simulink model "Embeddedsystem_Simulink"  (R2020a)
settings: Solver=FixedStepDiscrete  StartTime=0.0  StopTime=inf  FixedStep=0.1  RelTol=1e-3  EnableMultiTasking=on
libraries: frdmk64flib x4, simulink_extras x3, dspstat3 x1
settings Model: SimulationMode=external  ExtModeTrigDuration=5  Creator=luca9  LastModifiedBy=luca9
settings OptimizationCC: EnhancedBackFolding=on  PassReuseOutputArgsAs=Individual arguments  ZeroExternalMemoryAtStartup=off  ZeroInternalMemoryAtStartup=off  MaxStackSize=64  OptimizeBlockOrder=speed  DifferentSizesBufferReuse=on  OptimizationCustomize=off  EfficientTunableParamExpr=on
settings DebuggingCC: ParameterTunabilityLossMsg=error
settings HardwareCC: ProdBitPerPointer=32  ProdBitPerSizeT=32  ProdBitPerPtrDiffT=32  ProdLargestAtomicInteger=Long  ProdLargestAtomicFloat=Double  ProdWordSize=32  ProdHWDeviceType=ARM Compatible->ARM Cortex
settings SFSimCC: MATLABDynamicMemAlloc=off
settings RTWCC: SystemTargetFile=ert.tlc  HardwareBoard=NXP FRDM-K64F  TemplateMakefile=ert_default_tmf  GenerateReport=on  Toolchain=GNU Tools for ARM Embedded Processors
settings CodeAppCC: ForceParamTrailComments=on  IgnoreCustomStorageClasses=off  OperatorAnnotations=on  SimulinkDataObjDesc=on  SFDataObjDesc=on  InsertBlockDesc=on
settings ERTTargetCC: ExtMode=on  ExtModeTransport=4  ExtModeMexFile=sendToCommService  ExtModeMexArgs='sim_finalassignment' 0

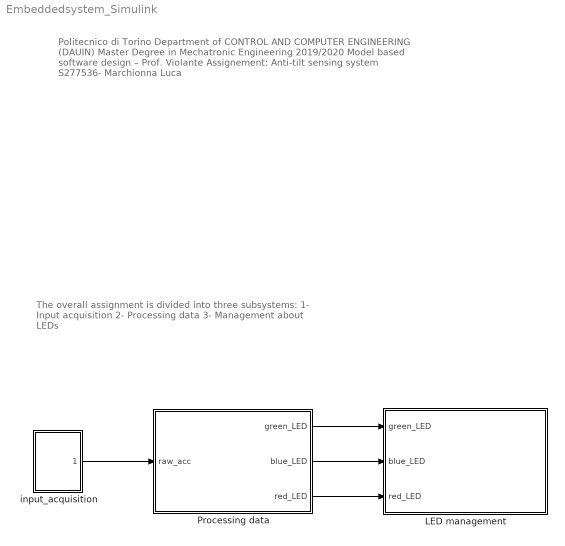
== system Embeddedsystem_Simulink ==
  note: The overall assignment is divided into three subsystems:
      | 1- Input acquisition
      | 2- Processing data
      | 3- Management about LEDs
  note: Politecnico di Torino
      | Department of CONTROL AND COMPUTER ENGINEERING (DAUIN)
      | Master Degree in Mechatronic Engineering
      | 2019/2020
      |
      | Model based software design – Prof. Violante
      | Assignement: Anti-tilt sensing system
      | S277536- Marchionna Luca
  " LED management" : Subsystem
  Processing data : Subsystem
  input_acquisition : Subsystem
  wires:
  input_acquisition/1(raw_acc) -> Processing data/1(raw_acc)
  Processing data/1(green_LED) -> " LED management"/1(green_LED)
  Processing data/2(blue_LED) -> " LED management"/2(blue_LED)
  Processing data/3(red_LED) -> " LED management"/3(red_LED)

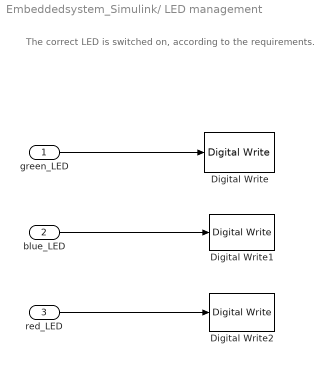
== system Embeddedsystem_Simulink/ LED management ==
  note: The correct LED is switched on, according to the requirements.
  green_LED : Inport
  blue_LED : Inport  Port=2
  red_LED : Inport  Port=3
  Digital Write : frdmk64flib/Digital Write  Whichpin=GREEN_LED
  Digital Write1 : frdmk64flib/Digital Write  Whichpin=BLUE_LED
  Digital Write2 : frdmk64flib/Digital Write  Whichpin=RED_LED
  wires:
  green_LED/1 -> Digital Write/1
  blue_LED/1 -> Digital Write1/1
  red_LED/1 -> Digital Write2/1

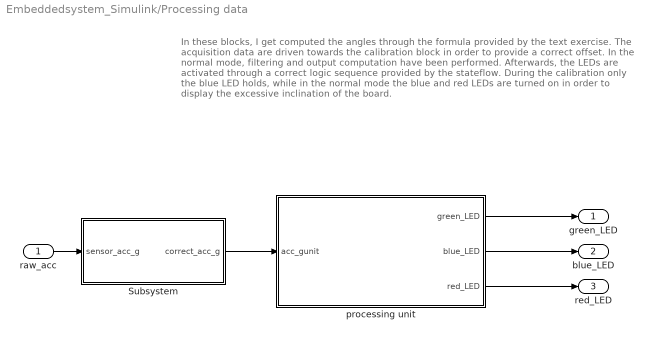
== system Embeddedsystem_Simulink/Processing data ==
  note: In these blocks, I get computed the angles through the formula provided by the text exercise. The acquisition data are driven towards the calibration block in order to provide a correct offset. In the normal mode, filtering and output computation have been performed.
      | Afterwards, the LEDs are activated through a correct logic sequence provided by the stateflow. During the calibration only the blue LED holds, while in the normal mode the blue and red LEDs are turned on in order to display the excessive inclination of the board.
  raw_acc : Inport
  Subsystem : Subsystem
  processing unit : Subsystem
  green_LED : Outport
  blue_LED : Outport  Port=2
  red_LED : Outport  Port=3
  wires:
  raw_acc/1 -> Subsystem/1(sensor_acc_g)
  Subsystem/1(correct_acc_g) -> processing unit/1(acc_gunit)
  processing unit/1(green_LED) -> green_LED/1
  processing unit/2(blue_LED) -> blue_LED/1
  processing unit/3(red_LED) -> red_LED/1

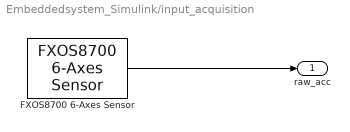
== system Embeddedsystem_Simulink/input_acquisition ==
  FXOS8700 6-Axes Sensor : frdmk64flib/FXOS8700 6-Axes Sensor  Activesensor=Accelerometer only  ODR=50Hz  HybridODR=400Hz  Accelfullrange=-2g to +2g  SampleTime=-1
  raw_acc : Outport
  wires:
  FXOS8700 6-Axes Sensor/1 -> raw_acc/1

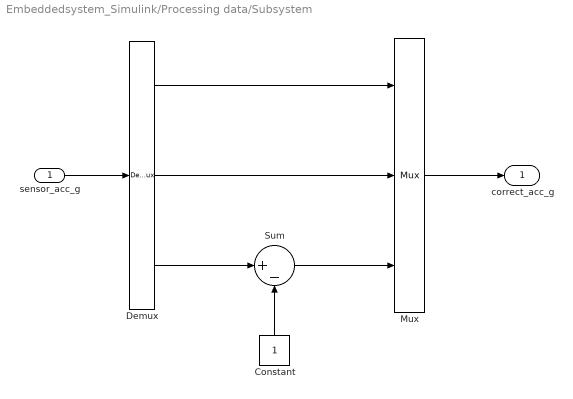
== system Embeddedsystem_Simulink/Processing data/Subsystem ==
  sensor_acc_g : Inport
  Constant : Constant
  Demux : Demux  Outputs=3
  Mux : Mux  Inputs=3
  Sum : Sum  Inputs=|+-
  correct_acc_g : Outport
  wires:
  sensor_acc_g/1 -> Demux/1
  Demux/3 -> Sum/1
  Mux/1 -> correct_acc_g/1
  Constant/1 -> Sum/2
  Demux/2 -> Mux/2
  Demux/1 -> Mux/1
  Sum/1 -> Mux/3

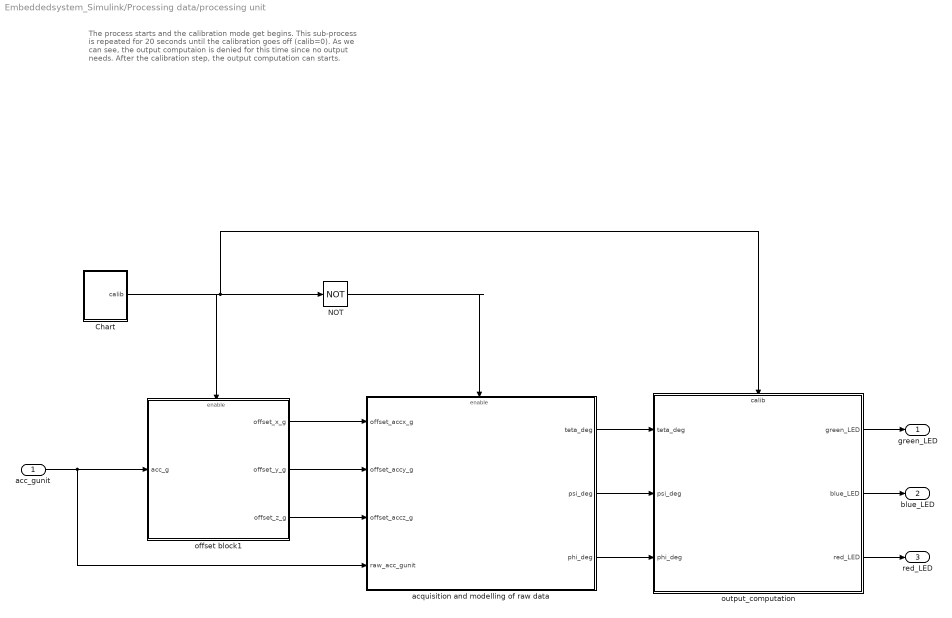
== system Embeddedsystem_Simulink/Processing data/processing unit ==
  note: The process starts and the calibration mode get begins. This sub-process is repeated for 20 seconds until the calibration goes off (calib=0). As we can see, the output computaion is denied for this time since no output needs. After the calibration step, the output computation can starts.
  acc_gunit : Inport
  Chart : Stateflow chart  TreatAsAtomicUnit=on
      settings: PortSchema="{\"entries\":[{\"content\":{\"sides\":[{\"content\":{\"connectorIds\":[]},\"type\":\"ConnectorPlacement.EquallySpacedRectSide\",\"uuid\":\"849f233e-f388-4235-a763-39289e6833f4\"},{\"content\":{\"connectorIds\":[],\"side\":\"RIGHT\"},\"type\":\"ConnectorPlacement.EquallySpacedRectSide\",\"uuid\":\"02f40bd9-b98f-494b-865f-ff408e26e3ae\"},{\"content\":{\"connectorIds\":[\"Out1\"],\"side\":\"TOP\"},\"type\":\"ConnectorPlacement.EquallySpacedRectSide\",\"uuid\":\"24d40e34-9a61-441c-a62a-e59ff23fe97d\"}]},\"type\":\"ConnectorPlacement.EquallySpacedConnector\",\"uuid\":\"996c4ffd-b183-49ea-a222-3899ee3ed888\"}],\"packageUris\":[\"http://schema.mathworks.com/mf0/Connector/19700101\"],\"version\":\"1.0\"}"
  NOT : Logic  Operator=NOT  IconShape=distinctive  AllPortsSameDT=off  OutDataTypeStr=boolean
  acquisition and modelling of raw data : Subsystem
  offset block1 : Subsystem
  output_computation : Subsystem
      settings: PortSchema="{\"entries\":[{\"content\":{\"sides\":[{\"content\":{\"connectorIds\":[\"In1\",\"In2\",\"In3\"]},\"type\":\"ConnectorPlacement.EquallySpacedRectSide\",\"uuid\":\"60aea4be-a06d-4eda-a7bc-981b750d10d1\"},{\"content\":{\"connectorIds\":[\"Out1\",\"Out2\",\"Out3\"],\"side\":\"RIGHT\"},\"type\":\"ConnectorPlacement.EquallySpacedRectSide\",\"uuid\":\"1715f949-f62d-450d-8914-9423294c064a\"},{\"content\":{\"connectorIds\":[\"In4\"],\"side\":\"TOP\"},\"type\":\"ConnectorPlacement.EquallySpacedRectSide\",\"uuid\":\"7760335e-0d5c-4cba-ab90-42ab2a2902db\"}]},\"type\":\"ConnectorPlacement.EquallySpacedConnector\",\"uuid\":\"a047fbe5-0454-4ad3-85fe-5a2833169652\"}],\"packageUris\":[\"http://schema.mathworks.com/mf0/Connector/19700101\"],\"version\":\"1.0\"}"
  green_LED : Outport
  blue_LED : Outport  Port=2
  red_LED : Outport  Port=3
  wires:
  acquisition and modelling of raw data/1(teta_deg) -> output_computation/1(teta_deg)
  Chart/1(calib) -> NOT/1, output_computation/4(calib), offset block1/Enable
  NOT/1 -> acquisition and modelling of raw data/Enable
  acc_gunit/1 -> acquisition and modelling of raw data/4(raw_acc_gunit), offset block1/1(acc_g)
  offset block1/1(offset_x_g) -> acquisition and modelling of raw data/1(offset_accx_g)
  offset block1/2(offset_y_g) -> acquisition and modelling of raw data/2(offset_accy_g)
  offset block1/3(offset_z_g) -> acquisition and modelling of raw data/3(offset_accz_g)
  acquisition and modelling of raw data/2(psi_deg) -> output_computation/2(psi_deg)
  acquisition and modelling of raw data/3(phi_deg) -> output_computation/3(phi_deg)
  output_computation/2(blue_LED) -> blue_LED/1
  output_computation/3(red_LED) -> red_LED/1
  output_computation/1(green_LED) -> green_LED/1

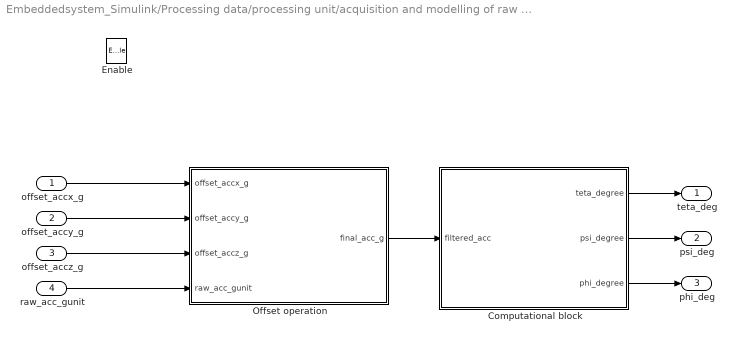
== system Embeddedsystem_Simulink/Processing data/processing unit/acquisition and modelling of raw data ==
  offset_accx_g : Inport
  offset_accy_g : Inport  Port=2
  offset_accz_g : Inport  Port=3
  raw_acc_gunit : Inport  Port=4
  Enable : EnablePort
  Computational block : Subsystem
  Offset operation : Subsystem
  teta_deg : Outport
  psi_deg : Outport  Port=2
  phi_deg : Outport  Port=3
  wires:
  offset_accx_g/1 -> Offset operation/1(offset_accx_g)
  offset_accz_g/1 -> Offset operation/3(offset_accz_g)
  Offset operation/1(final_acc_g) -> Computational block/1(filtered_acc)
  raw_acc_gunit/1 -> Offset operation/4(raw_acc_gunit)
  offset_accy_g/1 -> Offset operation/2(offset_accy_g)
  Computational block/1(teta_degree) -> teta_deg/1
  Computational block/3(phi_degree) -> phi_deg/1
  Computational block/2(psi_degree) -> psi_deg/1

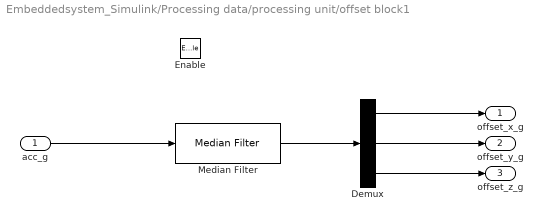
== system Embeddedsystem_Simulink/Processing data/processing unit/offset block1 ==
  acc_g : Inport
  Enable : EnablePort
  Demux : Demux  Outputs=3
  Median Filter : dspstat3/Median Filter  WindowLength=128  SimulateUsing=Interpreted execution
      settings: SourceProductBaseCode=DS
  offset_x_g : Outport
  offset_y_g : Outport  Port=2
  offset_z_g : Outport  Port=3
  wires:
  acc_g/1 -> Median Filter/1
  Demux/2 -> offset_y_g/1
  Median Filter/1 -> Demux/1
  Demux/1 -> offset_x_g/1
  Demux/3 -> offset_z_g/1

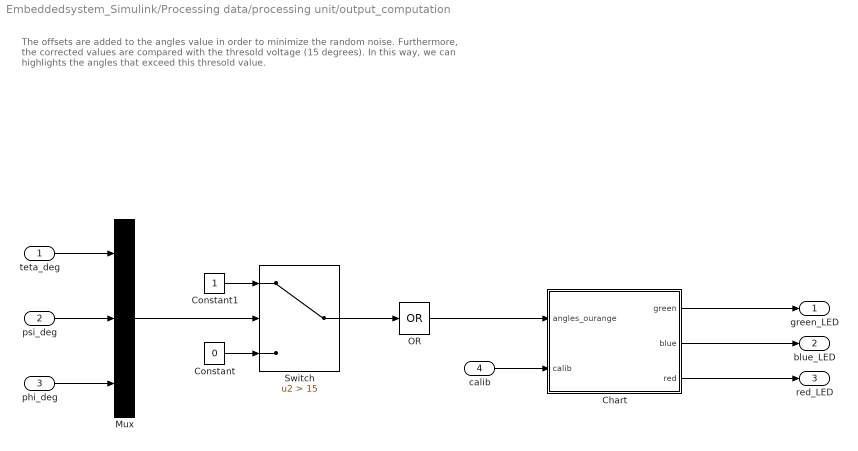
== system Embeddedsystem_Simulink/Processing data/processing unit/output_computation ==
  note: The offsets are added to the angles value in order to minimize the random noise. Furthermore, the corrected values are compared with the thresold voltage (15 degrees). In this way, we can highlights the angles that exceed this thresold value.
  teta_deg : Inport
  psi_deg : Inport  Port=2
  phi_deg : Inport  Port=3
  calib : Inport  Port=4
  Chart : Stateflow chart  TreatAsAtomicUnit=on
      settings: PortSchema="{\"entries\":[{\"content\":{\"sides\":[{\"content\":{\"connectorIds\":[\"In2\",\"In1\"]},\"type\":\"ConnectorPlacement.EquallySpacedRectSide\",\"uuid\":\"faf833d6-594c-410a-add6-5ce55fbfaff1\"},{\"content\":{\"connectorIds\":[\"Out1\",\"Out2\",\"Out3\"],\"side\":\"RIGHT\"},\"type\":\"ConnectorPlacement.EquallySpacedRectSide\",\"uuid\":\"c32c7775-d168-4cbd-91e2-7224e6ac9991\"},{\"content\":{\"connectorIds\":[],\"side\":\"TOP\"},\"type\":\"ConnectorPlacement.EquallySpacedRectSide\",\"uuid\":\"b777e44b-d9ef-458a-832d-3343b5e05232\"}]},\"type\":\"ConnectorPlacement.EquallySpacedConnector\",\"uuid\":\"539e4311-01e8-4a30-b4c5-5074bbcc3c5b\"}],\"packageUris\":[\"http://schema.mathworks.com/mf0/Connector/19700101\"],\"version\":\"1.0\"}"
  Constant : Constant  Value=0
  Constant1 : Constant
  Mux : Mux  Inputs=3
  OR : Logic  Operator=OR  Inputs=1  IconShape=distinctive  AllPortsSameDT=off  OutDataTypeStr=boolean
  Switch : Switch  Criteria=u2 > Threshold  Threshold=15
  green_LED : Outport
  blue_LED : Outport  Port=2
  red_LED : Outport  Port=3
  wires:
  Constant1/1 -> Switch/1
  Constant/1 -> Switch/3
  Switch/1 -> OR/1
  OR/1 -> Chart/2(angles_ourange)
  phi_deg/1 -> Mux/3
  psi_deg/1 -> Mux/2
  teta_deg/1 -> Mux/1
  Mux/1 -> Switch/2
  Chart/2(blue) -> blue_LED/1
  Chart/3(red) -> red_LED/1
  Chart/1(green) -> green_LED/1
  calib/1 -> Chart/1(calib)

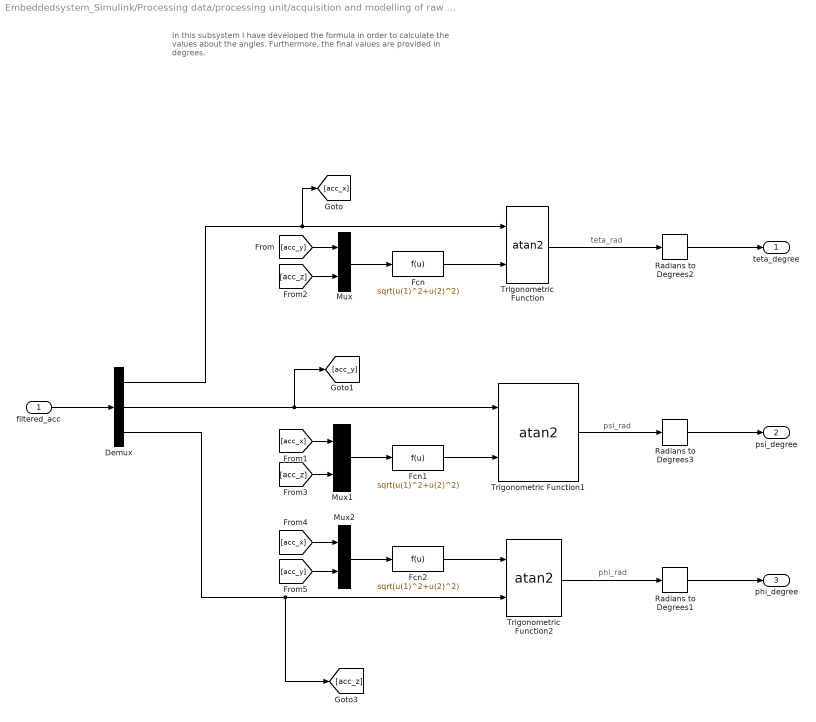
== system Embeddedsystem_Simulink/Processing data/processing unit/acquisition and modelling of raw data/Computational block ==
  note: phi_rad
  note: psi_rad
  note: teta_rad
  note: In this subsystem I have developed the formula in order to calculate the values about the angles. Furthermore, the final values are provided in degrees.
  filtered_acc : Inport
  Demux : Demux  Outputs=3
  Fcn : Fcn  Expr=sqrt(u(1)^2+u(2)^2)
  Fcn1 : Fcn  Expr=sqrt(u(1)^2+u(2)^2)
  Fcn2 : Fcn  Expr=sqrt(u(1)^2+u(2)^2)
  Mux : Mux  Inputs=2
  Mux1 : Mux  Inputs=2
  Mux2 : Mux  Inputs=2
  Radians to Degrees1 : simulink_extras/Transformations/Radians to Degrees
  Radians to Degrees2 : simulink_extras/Transformations/Radians to Degrees
  Radians to Degrees3 : simulink_extras/Transformations/Radians to Degrees
  Trigonometric Function : Trigonometry  Operator=atan2
  Trigonometric Function1 : Trigonometry  Operator=atan2
  Trigonometric Function2 : Trigonometry  Operator=atan2
  teta_degree : Outport
  psi_degree : Outport  Port=2
  phi_degree : Outport  Port=3
  wires:
  [acc_y] -> Mux2/2
  Mux/1 -> Fcn/1
  [acc_z] -> Mux1/2
  Mux1/1 -> Fcn1/1
  [acc_z] -> Mux/2
  Demux/2 -> [acc_y], Trigonometric Function1/1
  Mux2/1 -> Fcn2/1
  [acc_y] -> Mux/1
  Fcn1/1 -> Trigonometric Function1/2
  Demux/3 -> [acc_z], Trigonometric Function2/2
  [acc_x] -> Mux2/1
  [acc_x] -> Mux1/1
  Fcn2/1 -> Trigonometric Function2/1
  Fcn/1 -> Trigonometric Function/2
  Demux/1 -> [acc_x], Trigonometric Function/1
  filtered_acc/1 -> Demux/1
  Trigonometric Function/1 -> Radians to Degrees2/1
  Trigonometric Function1/1 -> Radians to Degrees3/1
  Trigonometric Function2/1 -> Radians to Degrees1/1
  Radians to Degrees2/1 -> teta_degree/1
  Radians to Degrees3/1 -> psi_degree/1
  Radians to Degrees1/1 -> phi_degree/1

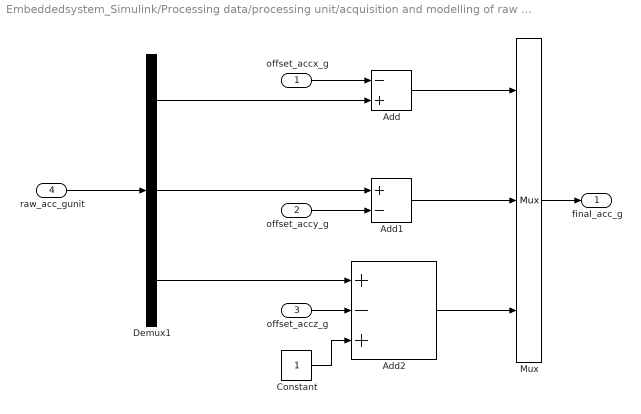
== system Embeddedsystem_Simulink/Processing data/processing unit/acquisition and modelling of raw data/Offset operation ==
  offset_accx_g : Inport
  offset_accy_g : Inport  Port=2
  offset_accz_g : Inport  Port=3
  raw_acc_gunit : Inport  Port=4
  Add : Sum  Inputs=-+
  Add1 : Sum  Inputs=+-
  Add2 : Sum  Inputs=+-+
  Constant : Constant
  Demux1 : Demux  Outputs=3
  Mux : Mux  Inputs=3
  final_acc_g : Outport
  wires:
  offset_accy_g/1 -> Add1/2
  offset_accx_g/1 -> Add/1
  offset_accz_g/1 -> Add2/2
  Demux1/2 -> Add1/1
  Demux1/3 -> Add2/1
  Demux1/1 -> Add/2
  raw_acc_gunit/1 -> Demux1/1
  Mux/1 -> final_acc_g/1
  Add1/1 -> Mux/2
  Add/1 -> Mux/1
  Constant/1 -> Add2/3
  Add2/1 -> Mux/3

== stateflow chart Embeddedsystem_Simulink/Processing data/processing unit/Chart ==
  state calibration
    en:
    calib=1;
  state calibration1
    en:
    calib=0;
  (default) -> calibration
  calibration -> calibration1 : after(20,sec)
  data: calib output

== stateflow chart Embeddedsystem_Simulink/Processing data/processing unit/output_computation/Chart ==
  state LED_inizialization
    en: blue=0;
    green=0;
    red=0;
  state LED_structureforcalibration
    en: blue=1;
    green=0;
    red=0;
  state LED_structureforinclination
    en: blue=0;
    state inclination_
      green=1;
      red=0;
    state warning1
      red=1;
      green=0;
    state no_warning
      red=0;
      green=1;
    (default) -> inclination_
    inclination_ -> warning1 [order 1] : [angles_ourange==1]
    inclination_ -> no_warning [order 2] : [angles_ourange==0]
    no_warning -> warning1 : [angles_ourange==1]
    warning1 -> no_warning : [angles_ourange==0]
  (default) -> LED_inizialization
  LED_inizialization -> LED_structureforcalibration : [calib==1]
  LED_structureforcalibration -> LED_structureforinclination : [calib==0]
  data: calib input; angles_ourange input; green output; blue output; red output
